simulink model "Boat_NonLinear_OL"  (R2020a)
settings: Solver=VariableStepAuto  StartTime=0.0  StopTime=10.0  RelTol=1e-3
settings Model: Creator=micro microndas  LastModifiedBy=micro microndas

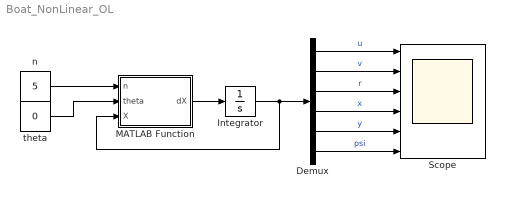
== system Boat_NonLinear_OL ==
  Demux : Demux  Outputs=6
  Integrator : Integrator  InitialCondition=[0 0 0 0 0 pi/4]
  MATLAB Function : MATLAB Function  TreatAsAtomicUnit=on
  Scope : Scope  NumInputPorts=6
  n : Constant  Value=5
  theta : Constant  Value=0
  wires:
  MATLAB Function/1(dX) -> Integrator/1
  Integrator/1 -> Demux/1, MATLAB Function/3(X)
  n/1 -> MATLAB Function/1(n)
  theta/1 -> MATLAB Function/2(theta)
  Demux/1 -> Scope/1  "u"
  Demux/2 -> Scope/2  "v"
  Demux/3 -> Scope/3  "r"
  Demux/4 -> Scope/4  "x"
  Demux/5 -> Scope/5  "y"
  Demux/6 -> Scope/6  "psi"

== matlab function Boat_NonLinear_OL/MATLAB Function ==
  data: n input; dX output; theta input; X input
function dX = fcn(n , theta, X)

 

%Parametros del sistema
m11 = 54;   m22 = 33.8;  m23 = 1.0115;  m32 = 1.0115;  m33 = 2.76; 
n11 = 15;   n22 = 7;     n23 = 23.8;    n32 = 0.1;     n33 = 1.095;
T1 = 0.26;  T2= 0.1; b = 1; 

 

%Calcular inversa de Matriz M

 

fu = (T1*abs(n)*n - T2*abs(n)*n*sqrt(X(1)^2 + (X(3)*b)^2) )*cos(theta);
fr = (T1*abs(n)*n - T2*abs(n)*n*sqrt(X(1)^2 + (X(3)*b)^2) )*sin(theta);

 

M_inv = [m11 0 0; 0 m22 m23 ; 0 m32 m33]^-1;
N = [ n11 0 0 ; 0 n22 n23 ; 0 n32 n33];

 

R = [cos(X(6)) -sin(X(6)) 0 ; sin(X(6)) cos(X(6)) 0; 0 0 1]*[ X(1); X(2); X(3)];

 

dX = [ M_inv*[fu; 0 ; fr*b] - M_inv*N*[X(1) ; X(2) ; X(3) ]; R];
